simulink model "controlmodel"  (R2016a)
settings: Solver=ode45  StartTime=0.0  StopTime=12.0  RelTol=1e-3
values from neighbouring files (symbols this model uses):
  gainBFL = 1    [LoadModel_dampedTM.m]
  gainBFP = 1    [LoadModel_dampedTM.m]
  gainBFR = 1    [LoadModel_dampedTM.m]
  gainBFT = 1    [LoadModel_dampedTM.m]
  gainBFV = 1    [LoadModel_dampedTM.m]
  gainBFY = 1    [LoadModel_dampedTM.m]
  gainGASBF = 1    [LoadModel_dampedTM.m]
  gainGASF0 = 1    [LoadModel_dampedTM.m]
  gainGASF1 = 1    [LoadModel_dampedTM.m]
  gainGASF2 = 1    [LoadModel_dampedTM.m]
  gainGASF3 = 1    [LoadModel_dampedTM.m]
  gainIML = 1    [LoadModel_dampedTM.m]
  gainIMP = 1    [LoadModel_dampedTM.m]
  gainIMR = 1    [LoadModel_dampedTM.m]
  gainIMT = 1    [LoadModel_dampedTM.m]
  gainIMV = 1    [LoadModel_dampedTM.m]
  gainIMY = 1    [LoadModel_dampedTM.m]
  gainIPL = 1    [LoadModel_dampedTM.m]
  gainIPT = 1    [LoadModel_dampedTM.m]
  gainIPY = 1    [LoadModel_dampedTM.m]
  gainLOCK_IML = 1    [LoadModel_dampedTM.m]
  gainLOCK_IMP = 1    [LoadModel_dampedTM.m]
  gainLOCK_IMY = 1    [LoadModel_dampedTM.m]
  gainMNL = 1    [LoadModel_dampedTM.m]
  gainMNLOCK_L = 1    [LoadModel_dampedTM.m]
  gainMNLOCK_P = 1    [LoadModel_dampedTM.m]
  gainMNLOCK_Y = 1    [LoadModel_dampedTM.m]
  gainMNP = 1    [LoadModel_dampedTM.m]
  gainMNR = 1    [LoadModel_dampedTM.m]
  gainMNT = 1    [LoadModel_dampedTM.m]
  gainMNV = 1    [LoadModel_dampedTM.m]
  gainMNY = 1    [LoadModel_dampedTM.m]
  gainOL_MNP = 1    [LoadModel_dampedTM.m]
  gainOL_MNY = 1    [LoadModel_dampedTM.m]
  gainTML = 1    [LoadModel_dampedTM.m]
  gainTML_LOCK = 0    [LoadModel_dampedTM.m]
  gainTMOL_IML = 1    [LoadModel_dampedTM.m]
  gainTMOL_IMP = 1    [LoadModel_dampedTM.m]
  gainTMOL_IMY = 1    [LoadModel_dampedTM.m]
  gainTMOL_MNL = 1    [LoadModel_dampedTM.m]
  gainTMOL_MNP = 1    [LoadModel_dampedTM.m]
  gainTMOL_MNY = 1    [LoadModel_dampedTM.m]
  gainTMP = 1    [LoadModel_dampedTM.m]
  gainTMY = 1    [LoadModel_dampedTM.m]
  Kopt_angle = 0.1    [LoadModel_dampedTM.m]
  Kopt_len = 0.1    [LoadModel_dampedTM.m]
  optic = 'ETMX'    [LoadModel_dampedTM.m]
undefined symbols (not defined in the file or in its folder): cMat_BF, cMat_IM, cMat_MN, cMat_TM, Filt, gain_actBFGAS, gain_actBFL, gain_actBFP, gain_actBFR, gain_actBFT, gain_actBFV, gain_actBFY, gain_actF0GAS, gain_actF1GAS, gain_actF2GAS, gain_actF3GAS, gain_actIML, gain_actIMP, gain_actIMR, gain_actIMT, gain_actIMV, gain_actIMY, gain_actIPL, gain_actIPT, gain_actIPY, gain_actMNL, gain_actMNP, gain_actMNR, gain_actMNT, gain_actMNV, gain_actMNY, gain_actTML, gain_actTMP, gain_actTMY, SW, sys1
libraries: cstblocks x49, LiveParts x49
(part 3 of 3)

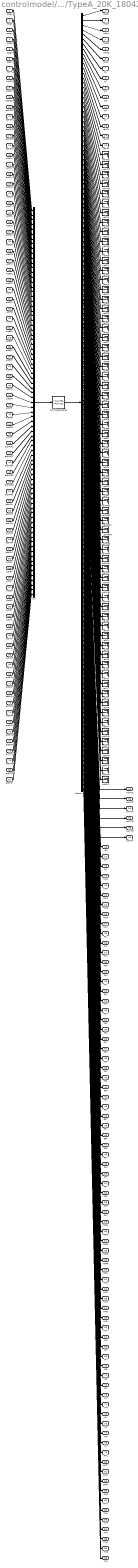
== system controlmodel/TypeA/Suspension/Suspension/TypeA_20K_180429 ==
  accgL : Inport
  accgT : Inport  Port=2
  accgV : Inport  Port=3
  accgR : Inport  Port=4
  accgP : Inport  Port=5
  accgY : Inport  Port=6
  actIPL : Inport  Port=7
  actIPT : Inport  Port=8
  actIPY : Inport  Port=9
  actMDL : Inport  Port=10
  actMDT : Inport  Port=11
  actMDV : Inport  Port=12
  actMDR : Inport  Port=13
  actMDP : Inport  Port=14
  actMDY : Inport  Port=15
  actF1L : Inport  Port=16
  actF1T : Inport  Port=17
  actF1V : Inport  Port=18
  actF1R : Inport  Port=19
  actF1P : Inport  Port=20
  actF1Y : Inport  Port=21
  actF2L : Inport  Port=22
  actF2T : Inport  Port=23
  actF2V : Inport  Port=24
  actF2R : Inport  Port=25
  actF2P : Inport  Port=26
  actF2Y : Inport  Port=27
  actF3L : Inport  Port=28
  actF3T : Inport  Port=29
  actF3V : Inport  Port=30
  actF3R : Inport  Port=31
  actF3P : Inport  Port=32
  actF3Y : Inport  Port=33
  actBFL : Inport  Port=34
  actBFT : Inport  Port=35
  actBFV : Inport  Port=36
  actBFR : Inport  Port=37
  actBFP : Inport  Port=38
  actBFY : Inport  Port=39
  actPFL : Inport  Port=40
  actPFT : Inport  Port=41
  actPFV : Inport  Port=42
  actPFR : Inport  Port=43
  actPFP : Inport  Port=44
  actPFY : Inport  Port=45
  actMNRL : Inport  Port=46
  actMNRT : Inport  Port=47
  actMNRV : Inport  Port=48
  actMNRR : Inport  Port=49
  actMNRP : Inport  Port=50
  actMNRY : Inport  Port=51
  actMNL : Inport  Port=52
  actMNT : Inport  Port=53
  actMNV : Inport  Port=54
  actMNR : Inport  Port=55
  actMNP : Inport  Port=56
  actMNY : Inport  Port=57
  actIRL : Inport  Port=58
  actIRT : Inport  Port=59
  actIRV : Inport  Port=60
  actIRR : Inport  Port=61
  actIRP : Inport  Port=62
  actIRY : Inport  Port=63
  actIML : Inport  Port=64
  actIMT : Inport  Port=65
  actIMV : Inport  Port=66
  actIMR : Inport  Port=67
  actIMP : Inport  Port=68
  actIMY : Inport  Port=69
  actRML : Inport  Port=70
  actRMT : Inport  Port=71
  actRMV : Inport  Port=72
  actRMR : Inport  Port=73
  actRMP : Inport  Port=74
  actRMY : Inport  Port=75
  actTML : Inport  Port=76
  actTMT : Inport  Port=77
  actTMV : Inport  Port=78
  actTMR : Inport  Port=79
  actTMP : Inport  Port=80
  actTMY : Inport  Port=81
  SAS State-Space : StateSpace  A=sys1.A  B=sys1.B  C=sys1.C  D=sys1.D  X0=0  ContinuousStateAttributes='SUS_SS_MODEL'
  demux : Demux  Outputs=162
  mux : Mux  Inputs=81
  velBFL : Terminator
  velBFP : Terminator
  velBFR : Terminator
  velBFT : Terminator
  velBFV : Terminator
  velBFY : Terminator
  velF1L : Terminator
  velF1P : Terminator
  velF1R : Terminator
  velF1T : Terminator
  velF1V : Terminator
  velF1Y : Terminator
  velF2L : Terminator
  velF2P : Terminator
  velF2R : Terminator
  velF2T : Terminator
  velF2V : Terminator
  velF2Y : Terminator
  velF3L : Terminator
  velF3P : Terminator
  velF3R : Terminator
  velF3T : Terminator
  velF3V : Terminator
  velF3Y : Terminator
  velIML : Terminator
  velIMP : Terminator
  velIMR : Terminator
  velIMT : Terminator
  velIMV : Terminator
  velIMY : Terminator
  velIRL : Terminator
  velIRP : Terminator
  velIRR : Terminator
  velIRT : Terminator
  velIRV : Terminator
  velIRY : Terminator
  velMDL : Terminator
  velMDP : Terminator
  velMDR : Terminator
  velMDT : Terminator
  velMDV : Terminator
  velMDY : Terminator
  velMNL : Terminator
  velMNP : Terminator
  velMNR : Terminator
  velMNRL : Terminator
  velMNRP : Terminator
  velMNRR : Terminator
  velMNRT : Terminator
  velMNRV : Terminator
  velMNRY : Terminator
  velMNT : Terminator
  velMNV : Terminator
  velMNY : Terminator
  velPFL : Terminator
  velPFP : Terminator
  velPFR : Terminator
  velPFT : Terminator
  velPFV : Terminator
  velPFY : Terminator
  velRML : Terminator
  velRMP : Terminator
  velRMR : Terminator
  velRMT : Terminator
  velRMV : Terminator
  velRMY : Terminator
  velgL : Outport
  velgT : Outport  Port=2
  velgV : Outport  Port=3
  velgR : Outport  Port=4
  velPg : Outport  Port=5
  velgY : Outport  Port=6
  gL : Outport  Port=7
  gT : Outport  Port=8
  gV : Outport  Port=9
  gR : Outport  Port=10
  gP : Outport  Port=11
  gY : Outport  Port=12
  velIPL : Outport  Port=13
  velIPT : Outport  Port=14
  velIPY : Outport  Port=15
  IPL : Outport  Port=16
  IPT : Outport  Port=17
  IPY : Outport  Port=18
  MDL : Outport  Port=19
  MDT : Outport  Port=20
  MDV : Outport  Port=21
  MDR : Outport  Port=22
  MDP : Outport  Port=23
  MDY : Outport  Port=24
  F1L : Outport  Port=25
  F1T : Outport  Port=26
  F1V : Outport  Port=27
  F1R : Outport  Port=28
  F1P : Outport  Port=29
  F1Y : Outport  Port=30
  F2L : Outport  Port=31
  F2T : Outport  Port=32
  F2V : Outport  Port=33
  F2R : Outport  Port=34
  F2P : Outport  Port=35
  F2Y : Outport  Port=36
  F3L : Outport  Port=37
  F3T : Outport  Port=38
  F3V : Outport  Port=39
  F3R : Outport  Port=40
  F3P : Outport  Port=41
  F3Y : Outport  Port=42
  BFL : Outport  Port=43
  BFT : Outport  Port=44
  BFV : Outport  Port=45
  BFR : Outport  Port=46
  BFP : Outport  Port=47
  BFY : Outport  Port=48
  PFL : Outport  Port=49
  PFT : Outport  Port=50
  PFV : Outport  Port=51
  PFR : Outport  Port=52
  PFP : Outport  Port=53
  PFY : Outport  Port=54
  MNRL : Outport  Port=55
  MNRT : Outport  Port=56
  MNRV : Outport  Port=57
  MNRR : Outport  Port=58
  MNRP : Outport  Port=59
  MNRY : Outport  Port=60
  MNL : Outport  Port=61
  MNT : Outport  Port=62
  MNV : Outport  Port=63
  MNR : Outport  Port=64
  MNP : Outport  Port=65
  MNY : Outport  Port=66
  IRL : Outport  Port=67
  IRT : Outport  Port=68
  IRV : Outport  Port=69
  IRR : Outport  Port=70
  IRP : Outport  Port=71
  IRY : Outport  Port=72
  IML : Outport  Port=73
  IMT : Outport  Port=74
  IMV : Outport  Port=75
  IMR : Outport  Port=76
  IMP : Outport  Port=77
  IMY : Outport  Port=78
  RML : Outport  Port=79
  RMT : Outport  Port=80
  RMV : Outport  Port=81
  RMR : Outport  Port=82
  RMP : Outport  Port=83
  RMY : Outport  Port=84
  TML : Outport  Port=85
  TMT : Outport  Port=86
  TMV : Outport  Port=87
  TMR : Outport  Port=88
  TMP : Outport  Port=89
  TMY : Outport  Port=90
  velTML : Outport  Port=91
  velTMT : Outport  Port=92
  velTMV : Outport  Port=93
  velTMR : Outport  Port=94
  velTMP : Outport  Port=95
  velTMY : Outport  Port=96
  wires:
  mux/1 -> SAS State-Space/1
  SAS State-Space/1 -> demux/1
  accgL/1 -> mux/1
  accgT/1 -> mux/2
  accgV/1 -> mux/3
  accgR/1 -> mux/4
  accgP/1 -> mux/5
  accgY/1 -> mux/6
  actIPL/1 -> mux/7
  actIPT/1 -> mux/8
  actIPY/1 -> mux/9
  actMDL/1 -> mux/10
  actMDT/1 -> mux/11
  actMDV/1 -> mux/12
  actMDR/1 -> mux/13
  actMDP/1 -> mux/14
  actMDY/1 -> mux/15
  actF1L/1 -> mux/16
  actF1T/1 -> mux/17
  actF1V/1 -> mux/18
  actF1R/1 -> mux/19
  actF1P/1 -> mux/20
  actF1Y/1 -> mux/21
  actF2L/1 -> mux/22
  actF2T/1 -> mux/23
  actF2V/1 -> mux/24
  actF2R/1 -> mux/25
  actF2P/1 -> mux/26
  actF2Y/1 -> mux/27
  actF3L/1 -> mux/28
  actF3T/1 -> mux/29
  actF3V/1 -> mux/30
  actF3R/1 -> mux/31
  actF3P/1 -> mux/32
  actF3Y/1 -> mux/33
  actBFL/1 -> mux/34
  actBFT/1 -> mux/35
  actBFV/1 -> mux/36
  actBFR/1 -> mux/37
  actBFP/1 -> mux/38
  actBFY/1 -> mux/39
  actPFL/1 -> mux/40
  actPFT/1 -> mux/41
  actPFV/1 -> mux/42
  actPFR/1 -> mux/43
  actPFP/1 -> mux/44
  actPFY/1 -> mux/45
  actMNRL/1 -> mux/46
  actMNRT/1 -> mux/47
  actMNRV/1 -> mux/48
  actMNRR/1 -> mux/49
  actMNRP/1 -> mux/50
  actMNRY/1 -> mux/51
  actMNL/1 -> mux/52
  actMNT/1 -> mux/53
  actMNV/1 -> mux/54
  actMNR/1 -> mux/55
  actMNP/1 -> mux/56
  actMNY/1 -> mux/57
  actIRL/1 -> mux/58
  actIRT/1 -> mux/59
  actIRV/1 -> mux/60
  actIRR/1 -> mux/61
  actIRP/1 -> mux/62
  actIRY/1 -> mux/63
  actIML/1 -> mux/64
  actIMT/1 -> mux/65
  actIMV/1 -> mux/66
  actIMR/1 -> mux/67
  actIMP/1 -> mux/68
  actIMY/1 -> mux/69
  actRML/1 -> mux/70
  actRMT/1 -> mux/71
  actRMV/1 -> mux/72
  actRMR/1 -> mux/73
  actRMP/1 -> mux/74
  actRMY/1 -> mux/75
  actTML/1 -> mux/76
  actTMT/1 -> mux/77
  actTMV/1 -> mux/78
  actTMR/1 -> mux/79
  actTMP/1 -> mux/80
  actTMY/1 -> mux/81
  demux/1 -> velgL/1
  demux/2 -> velgT/1
  demux/3 -> velgV/1
  demux/4 -> velgR/1
  demux/5 -> velPg/1
  demux/6 -> velgY/1
  demux/7 -> gL/1
  demux/8 -> gT/1
  demux/9 -> gV/1
  demux/10 -> gR/1
  demux/11 -> gP/1
  demux/12 -> gY/1
  demux/13 -> velIPL/1
  demux/14 -> velIPT/1
  demux/15 -> velIPY/1
  demux/16 -> velMDL/1
  demux/17 -> velMDT/1
  demux/18 -> velMDV/1
  demux/19 -> velMDR/1
  demux/20 -> velMDP/1
  demux/21 -> velMDY/1
  demux/22 -> velF1L/1
  demux/23 -> velF1T/1
  demux/24 -> velF1V/1
  demux/25 -> velF1R/1
  demux/26 -> velF1P/1
  demux/27 -> velF1Y/1
  demux/28 -> velF2L/1
  demux/29 -> velF2T/1
  demux/30 -> velF2V/1
  demux/31 -> velF2R/1
  demux/32 -> velF2P/1
  demux/33 -> velF2Y/1
  demux/34 -> velF3L/1
  demux/35 -> velF3T/1
  demux/36 -> velF3V/1
  demux/37 -> velF3R/1
  demux/38 -> velF3P/1
  demux/39 -> velF3Y/1
  demux/40 -> velBFL/1
  demux/41 -> velBFT/1
  demux/42 -> velBFV/1
  demux/43 -> velBFR/1
  demux/44 -> velBFP/1
  demux/45 -> velBFY/1
  demux/46 -> velPFL/1
  demux/47 -> velPFT/1
  demux/48 -> velPFV/1
  demux/49 -> velPFR/1
  demux/50 -> velPFP/1
  demux/51 -> velPFY/1
  demux/52 -> velMNRL/1
  demux/53 -> velMNRT/1
  demux/54 -> velMNRV/1
  demux/55 -> velMNRR/1
  demux/56 -> velMNRP/1
  demux/57 -> velMNRY/1
  demux/58 -> velMNL/1
  demux/59 -> velMNT/1
  demux/60 -> velMNV/1
  demux/61 -> velMNR/1
  demux/62 -> velMNP/1
  demux/63 -> velMNY/1
  demux/64 -> velIRL/1
  demux/65 -> velIRT/1
  demux/66 -> velIRV/1
  demux/67 -> velIRR/1
  demux/68 -> velIRP/1
  demux/69 -> velIRY/1
  demux/70 -> velIML/1
  demux/71 -> velIMT/1
  demux/72 -> velIMV/1
  demux/73 -> velIMR/1
  demux/74 -> velIMP/1
  demux/75 -> velIMY/1
  demux/76 -> velRML/1
  demux/77 -> velRMT/1
  demux/78 -> velRMV/1
  demux/79 -> velRMR/1
  demux/80 -> velRMP/1
  demux/81 -> velRMY/1
  demux/82 -> velTML/1
  demux/83 -> velTMT/1
  demux/84 -> velTMV/1
  demux/85 -> velTMR/1
  demux/86 -> velTMP/1
  demux/87 -> velTMY/1
  demux/88 -> IPL/1
  demux/89 -> IPT/1
  demux/90 -> IPY/1
  demux/91 -> MDL/1
  demux/92 -> MDT/1
  demux/93 -> MDV/1
  demux/94 -> MDR/1
  demux/95 -> MDP/1
  demux/96 -> MDY/1
  demux/97 -> F1L/1
  demux/98 -> F1T/1
  demux/99 -> F1V/1
  demux/100 -> F1R/1
  demux/101 -> F1P/1
  demux/102 -> F1Y/1
  demux/103 -> F2L/1
  demux/104 -> F2T/1
  demux/105 -> F2V/1
  demux/106 -> F2R/1
  demux/107 -> F2P/1
  demux/108 -> F2Y/1
  demux/109 -> F3L/1
  demux/110 -> F3T/1
  demux/111 -> F3V/1
  demux/112 -> F3R/1
  demux/113 -> F3P/1
  demux/114 -> F3Y/1
  demux/115 -> BFL/1
  demux/116 -> BFT/1
  demux/117 -> BFV/1
  demux/118 -> BFR/1
  demux/119 -> BFP/1
  demux/120 -> BFY/1
  demux/121 -> PFL/1
  demux/122 -> PFT/1
  demux/123 -> PFV/1
  demux/124 -> PFR/1
  demux/125 -> PFP/1
  demux/126 -> PFY/1
  demux/127 -> MNRL/1
  demux/128 -> MNRT/1
  demux/129 -> MNRV/1
  demux/130 -> MNRR/1
  demux/131 -> MNRP/1
  demux/132 -> MNRY/1
  demux/133 -> MNL/1
  demux/134 -> MNT/1
  demux/135 -> MNV/1
  demux/136 -> MNR/1
  demux/137 -> MNP/1
  demux/138 -> MNY/1
  demux/139 -> IRL/1
  demux/140 -> IRT/1
  demux/141 -> IRV/1
  demux/142 -> IRR/1
  demux/143 -> IRP/1
  demux/144 -> IRY/1
  demux/145 -> IML/1
  demux/146 -> IMT/1
  demux/147 -> IMV/1
  demux/148 -> IMR/1
  demux/149 -> IMP/1
  demux/150 -> IMY/1
  demux/151 -> RML/1
  demux/152 -> RMT/1
  demux/153 -> RMV/1
  demux/154 -> RMR/1
  demux/155 -> RMP/1
  demux/156 -> RMY/1
  demux/157 -> TML/1
  demux/158 -> TMT/1
  demux/159 -> TMV/1
  demux/160 -> TMR/1
  demux/161 -> TMP/1
  demux/162 -> TMY/1
